simulink model "GetData"  (R2022b)
settings: Solver=VariableStepAuto  StartTime=0.0  StopTime=48  RelTol=1e-3
settings Model: Creator=jim  LastModifiedBy=jim

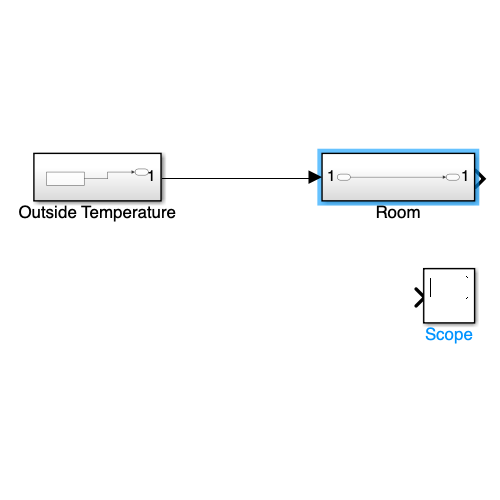
[thumbnail: Simulink's stored preview of the top-level diagram]
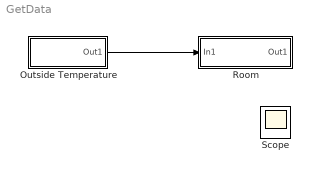
== system GetData ==
  Outside Temperature : Subsystem
  Room : Subsystem
  Scope : Scope
  wires:
  Outside Temperature/1(Out1) -> Room/1(In1)

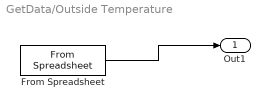
== system GetData/Outside Temperature ==
  From Spreadsheet : FromSpreadsheet  FileName=/Users/jim/Dropbox/GitHub Clones/CT549/code/04_Lecture/01 Get Data/aimsir17.xlsx
  Out1 : Outport
  wires:
  From Spreadsheet/1 -> Out1/1

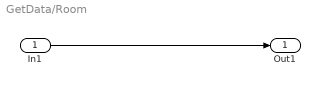
== system GetData/Room ==
  In1 : Inport
  Out1 : Outport
  wires:
  In1/1 -> Out1/1
